simulink model "Dyn_PointMass_R2015B"  (R2015b)
settings: Solver=ode4  SolverMode=SingleTasking  StartTime=0.0  StopTime=simInit.TSIM  FixedStep=simInit.dt  MaxStep=simInit.dt  RelTol=1e-3
InitFcn:
  | close all
undefined symbols (not defined in the file): base_windspeed, constr, DE2019, DiscIntNeverNeededParam, ENVMT, Lbooth, loiterStates, params, simInit, T, winchParameter
libraries: simulink x40, simulink_extras x3, dspsigops x1
(part 2 of 5)

== system Dyn_PointMass_R2015B/WinchControl_SS_6/WinchDynamics ==
  for_tether_tot : Inport
  control_moments : Inport  Port=2
  Discrete-Time Integrator : DiscreteIntegrator  InitialCondition=winchParameter.lj_dot_init  InitialConditionSetting=State (most efficient)  SampleTime=-1  LimitOutput=on  UpperSaturationLimit=constr.winchParameter.v_max/winchParameter.radius  LowerSaturationLimit=constr.winchParameter.v_min/winchParameter.radius  ICPrevOutput=DiscIntNeverNeededParam  ICPrevScaledInput=DiscIntNeverNeededParam
  FrictionCoefficient : Gain  Gain=winchParameter.friction
  Gain{,2..6} (6 alike) : Gain  Gain=winchParameter.radius
  Gain1 : Gain  Gain=1/winchParameter.inertia
  Integrator : Integrator  InitialCondition=winchParameter.winch_angle_init
  Saturation1 : Saturate  UpperLimit=constr.winchParameter.a_max/winchParameter.radius  LowerLimit=constr.winchParameter.a_min/winchParameter.radius
  Sum : Sum  Inputs=+-+
  winch acc : Scope  NumInputPorts=2
  tether_length : Outport
  theta_dot : Outport  Port=2
  winch_acc : Outport  Port=3
  winch_vel : Outport  Port=4
  wires:
  Gain/1 -> tether_length/1
  Gain2/1 -> Sum/1
  Sum/1 -> Gain1/1
  Integrator/1 -> Gain/1  "winch_angle"
  Discrete-Time Integrator/1 -> Gain4/1, FrictionCoefficient/1, theta_dot/1, Integrator/1  "winch_angVel"
  control_moments/1 -> Sum/3
  FrictionCoefficient/1 -> Sum/2
  for_tether_tot/1 -> Gain2/1
  Gain1/1 -> Saturation1/1, Gain5/1, Gain3/1
  Saturation1/1 -> Discrete-Time Integrator/1, Gain6/1  "omega_dot"
  Gain4/1 -> winch_vel/1
  Gain3/1 -> winch_acc/1
  Gain5/1 -> winch acc/1
  Gain6/1 -> winch acc/2

== system Dyn_PointMass_R2015B/AirborneSystem/AttitudeDynamics/SecondOrderReferenceModel_alpha_a ==
  y_cmd : Inport
  Constant : Constant  Value=omega0_max
  Discrete-Time Integrator : DiscreteIntegrator  InitialConditionSetting=State (most efficient)  SampleTime=-1  LimitOutput=on  UpperSaturationLimit=y_max  LowerSaturationLimit=y_min  ICPrevOutput=DiscIntNeverNeededParam  ICPrevScaledInput=DiscIntNeverNeededParam
  Discrete-Time Integrator1 : DiscreteIntegrator  InitialConditionSetting=State (most efficient)  SampleTime=-1  LimitOutput=on  UpperSaturationLimit=yd_max  LowerSaturationLimit=yd_min  ICPrevOutput=DiscIntNeverNeededParam  ICPrevScaledInput=DiscIntNeverNeededParam
  Gain2 : Gain  Gain=2*zeta0
  Product : Product  Inputs=3
  Product1 : Product
  Saturation : Saturate  UpperLimit=y_max  LowerLimit=y_min
  Saturation1 : Saturate  UpperLimit=y2d_max  LowerLimit=y2d_min
  Sum : Sum  Inputs=|+-
  Sum1 : Sum  Inputs=|+-
  y_ref : Outport
  wires:
  Product1/1 -> Gain2/1
  Constant/1 -> Product1/2, Product/3, Product/1
  Product/1 -> Sum/1
  y_cmd/1 -> Saturation/1
  Discrete-Time Integrator1/1 -> Discrete-Time Integrator/1, Product1/1
  Sum/1 -> Saturation1/1
  Gain2/1 -> Sum/2
  Sum1/1 -> Product/2
  Saturation1/1 -> Discrete-Time Integrator1/1
  Saturation/1 -> Sum1/1
  Discrete-Time Integrator/1 -> y_ref/1, Sum1/2

== system Dyn_PointMass_R2015B/AirborneSystem/AttitudeDynamics/SecondOrderReferenceModel_mu_a ==
  y_cmd : Inport
  Constant : Constant  Value=omega0_max
  Discrete-Time Integrator : DiscreteIntegrator  InitialConditionSetting=State (most efficient)  SampleTime=-1  LimitOutput=on  UpperSaturationLimit=y_max  LowerSaturationLimit=y_min  ICPrevOutput=DiscIntNeverNeededParam  ICPrevScaledInput=DiscIntNeverNeededParam
  Discrete-Time Integrator1 : DiscreteIntegrator  InitialConditionSetting=State (most efficient)  SampleTime=-1  LimitOutput=on  UpperSaturationLimit=yd_max  LowerSaturationLimit=yd_min  ICPrevOutput=DiscIntNeverNeededParam  ICPrevScaledInput=DiscIntNeverNeededParam
  Gain2 : Gain  Gain=2*zeta0
  Product : Product  Inputs=3
  Product1 : Product
  Saturation : Saturate  UpperLimit=y_max  LowerLimit=y_min
  Saturation1 : Saturate  UpperLimit=y2d_max  LowerLimit=y2d_min
  Sum : Sum  Inputs=|+-
  Sum1 : Sum  Inputs=|+-
  y_ref : Outport
  wires:
  Product1/1 -> Gain2/1
  Constant/1 -> Product1/2, Product/3, Product/1
  Product/1 -> Sum/1
  y_cmd/1 -> Saturation/1
  Discrete-Time Integrator1/1 -> Discrete-Time Integrator/1, Product1/1
  Sum/1 -> Saturation1/1
  Gain2/1 -> Sum/2
  Sum1/1 -> Product/2
  Saturation1/1 -> Discrete-Time Integrator1/1
  Saturation/1 -> Sum1/1
  Discrete-Time Integrator/1 -> y_ref/1, Sum1/2

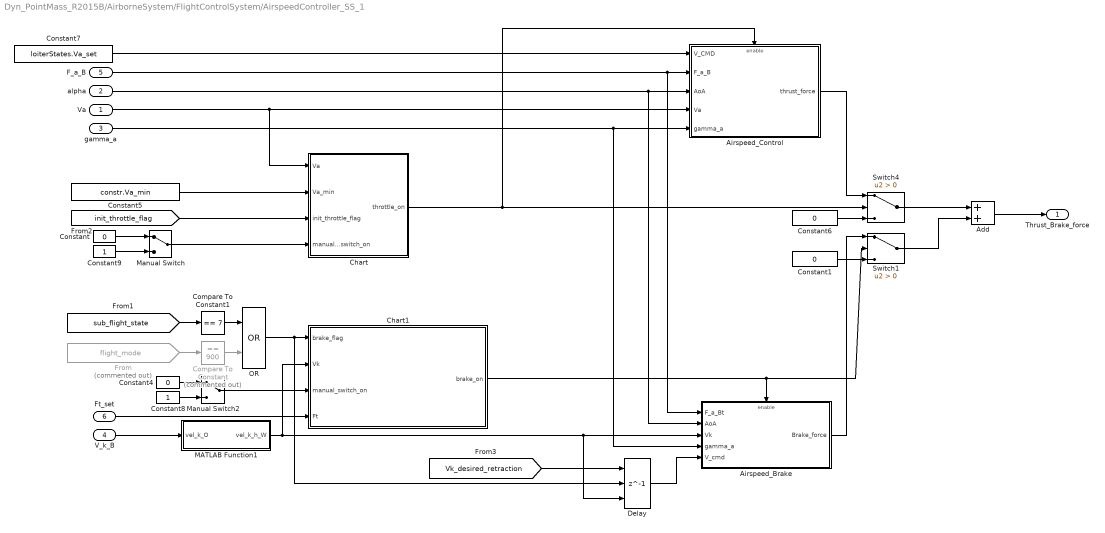
== system Dyn_PointMass_R2015B/AirborneSystem/FlightControlSystem/AirspeedController_SS_1 ==
  Va : Inport
  alpha : Inport  Port=2
  gamma_a : Inport  Port=3
  V_k_B : Inport  Port=4
  F_a_B : Inport  Port=5
  Ft_set : Inport  Port=6
  Add : Sum
  Airspeed_Brake : Subsystem
  Airspeed_Control : Subsystem
  Chart : Stateflow chart  TreatAsAtomicUnit=on
  Chart1 : Stateflow chart  TreatAsAtomicUnit=on  mask{Ft_retract=params.F_t_retraction_set*params.F_t_traction_set, Vk_min=30}
      mask prompts: Ft_retract "Retraction force"; Vk_min "Minimum Vk"
  Compare To Constant : simulink/Logic and Bit Operations/Compare To Constant  Commented=on  relop===  const=900  OutDataTypeStr=boolean
  Compare To Constant1 : simulink/Logic and Bit Operations/Compare To Constant  relop===  const=7  OutDataTypeStr=boolean
  Constant{,1,4,6} (4 alike) : Constant  Value=0
  Constant5 : Constant  Value=constr.Va_min
  Constant7 : Constant  Value=loiterStates.Va_set
  Constant8 : Constant
  Constant9 : Constant
  Delay : Delay  DelayLength=1  InitialConditionSource=Input port  ExternalReset=Rising
      settings: InputPortMap=u0,r5,p4
  From : From  Commented=on  GotoTag=flight_mode  TagVisibility=global
  MATLAB Function1 : MATLAB Function  TreatAsAtomicUnit=on
  Manual Switch : ManualSwitch
  Manual Switch2 : ManualSwitch
  OR : Logic  Operator=OR  IconShape=distinctive  AllPortsSameDT=off  OutDataTypeStr=boolean
  Switch1 : Switch  Criteria=u2 > Threshold
  Switch4 : Switch  Criteria=u2 > Threshold
  Thrust_Brake_force : Outport
  wires:
  Switch1/1 -> Add/2
  Constant1/1 -> Switch1/3
  [Vk_desired_retraction] -> Delay/1
  Compare To Constant/1 -> OR/2
  Compare To Constant1/1 -> OR/1
  MATLAB Function1/1(vel_k_h_W) -> Chart1/2(Vk), Delay/3, Airspeed_Brake/3(Vk)
  V_k_B/1 -> MATLAB Function1/1(vel_k_O)
  Delay/1 -> Airspeed_Brake/5(V_cmd)
  Constant8/1 -> Manual Switch2/2
  Constant4/1 -> Manual Switch2/1
  Add/1 -> Thrust_Brake_force/1
  From/1 -> Compare To Constant/1
  [sub_flight_state] -> Compare To Constant1/1
  OR/1 -> Chart1/1(brake_flag), Delay/2
  Manual Switch2/1 -> Chart1/3(manual_switch_on)
  Ft_set/1 -> Chart1/4(Ft)
  Airspeed_Brake/1(Brake_force) -> Switch1/1
  Chart1/1(brake_on) -> Switch1/2, Airspeed_Brake/Enable
  Airspeed_Control/1(thrust_force) -> Switch4/1
  Constant5/1 -> Chart/2(Va_min)
  Va/1 -> Chart/1(Va), Airspeed_Control/4(Va)
  Chart/1(throttle_on) -> Switch4/2, Airspeed_Control/Enable
  Constant9/1 -> Manual Switch/2
  [init_throttle_flag] -> Chart/3(init_throttle_flag)
  alpha/1 -> Airspeed_Control/3(AoA), Airspeed_Brake/2(AoA)
  Constant7/1 -> Airspeed_Control/1(V_CMD)
  Manual Switch/1 -> Chart/4(manual_switch_on)
  Constant/1 -> Manual Switch/1
  Constant6/1 -> Switch4/3
  F_a_B/1 -> Airspeed_Control/2(F_a_B), Airspeed_Brake/1(F_a_Bt)
  gamma_a/1 -> Airspeed_Control/5(gamma_a), Airspeed_Brake/4(gamma_a)
  Switch4/1 -> Add/1

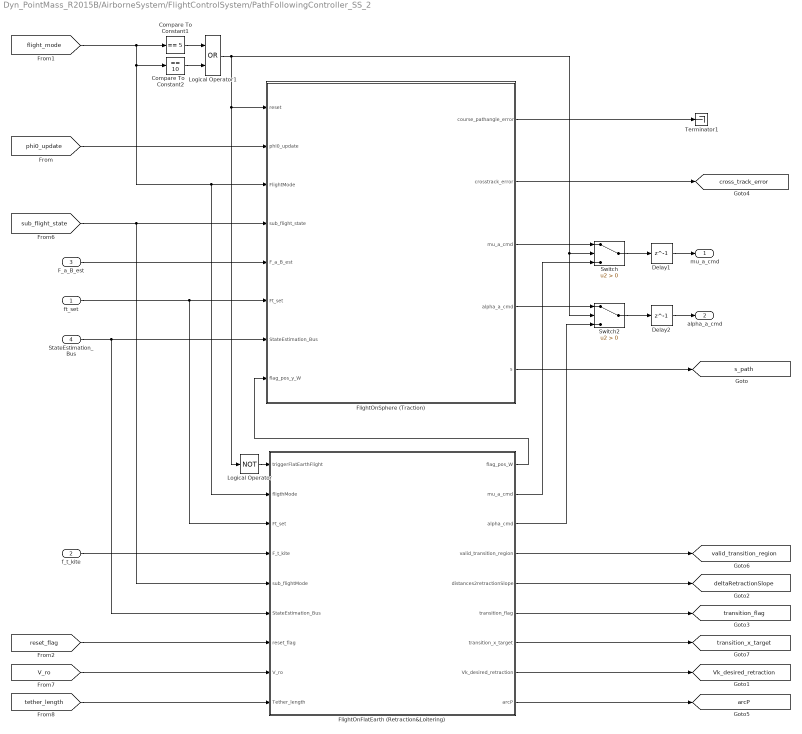
== system Dyn_PointMass_R2015B/AirborneSystem/FlightControlSystem/PathFollowingController_SS_2 ==
  ft_set : Inport
  f_t_kite : Inport  Port=2
  F_a_B_est : Inport  Port=3  PortDimensions=[3,1]
  StateEstimation_Bus : Inport  Port=4
  Compare To Constant1 : simulink/Logic and Bit Operations/Compare To Constant  relop===  const=5  OutDataTypeStr=boolean
  Compare To Constant2 : simulink/Logic and Bit Operations/Compare To Constant  relop===  const=10  OutDataTypeStr=boolean
  Delay1 : Delay  DelayLength=1
  Delay2 : Delay  DelayLength=1
  FlightOnFlatEarth (Retraction&Loitering) : Subsystem
  FlightOnSphere (Traction) : Subsystem
  Logical Operator : Logic  Operator=NOT  AllPortsSameDT=off  OutDataTypeStr=boolean
  Logical Operator1 : Logic  Operator=OR  AllPortsSameDT=off  OutDataTypeStr=boolean
  Switch : Switch  Criteria=u2 > Threshold
  Switch2 : Switch  Criteria=u2 > Threshold
  Terminator1 : Terminator
  mu_a_cmd : Outport  PortDimensions=1
  alpha_a_cmd : Outport  Port=2  PortDimensions=1
  tag scope: Vk_desired_retraction=global, arcP=global, cross_track_error=global, deltaRetractionSlope=global, s_path=global, transition_flag=global, transition_x_target=global, valid_transition_region=global
  wires:
  FlightOnFlatEarth (Retraction&Loitering)/9(arcP) -> [arcP]
  [sub_flight_state] -> FlightOnSphere (Traction)/4(sub_flight_state), FlightOnFlatEarth (Retraction&Loitering)/5(sub_flightMode)
  [tether_length] -> FlightOnFlatEarth (Retraction&Loitering)/9(Tether_length)
  [V_ro] -> FlightOnFlatEarth (Retraction&Loitering)/8(V_ro)
  FlightOnFlatEarth (Retraction&Loitering)/8(Vk_desired_retraction) -> [Vk_desired_retraction]
  FlightOnFlatEarth (Retraction&Loitering)/7(transition_x_target) -> [transition_x_target]
  FlightOnFlatEarth (Retraction&Loitering)/1(flag_pos_W) -> FlightOnSphere (Traction)/8(flag_pos_y_W)
  FlightOnFlatEarth (Retraction&Loitering)/5(distances2retractionSlope) -> [deltaRetractionSlope]
  [reset_flag] -> FlightOnFlatEarth (Retraction&Loitering)/7(reset_flag)
  FlightOnFlatEarth (Retraction&Loitering)/6(transition_flag) -> [transition_flag]
  [phi0_update] -> FlightOnSphere (Traction)/2(phi0_update)
  FlightOnSphere (Traction)/5(s) -> [s_path]
  Compare To Constant2/1 -> Logical Operator1/2
  Compare To Constant1/1 -> Logical Operator1/1
  [flight_mode] -> Compare To Constant2/1, FlightOnSphere (Traction)/3(FlightMode), FlightOnFlatEarth (Retraction&Loitering)/2(fligthMode), Compare To Constant1/1
  FlightOnSphere (Traction)/2(crosstrack_error) -> [cross_track_error]
  FlightOnSphere (Traction)/1(course_pathangle_error) -> Terminator1/1
  FlightOnSphere (Traction)/3(mu_a_cmd) -> Switch/1
  FlightOnSphere (Traction)/4(alpha_a_cmd) -> Switch2/1
  F_a_B_est/1 -> FlightOnSphere (Traction)/5(F_a_B_est)
  f_t_kite/1 -> FlightOnFlatEarth (Retraction&Loitering)/4(F_t_kite)
  Switch2/1 -> Delay2/1
  Switch/1 -> Delay1/1
  Delay1/1 -> mu_a_cmd/1
  Delay2/1 -> alpha_a_cmd/1
  ft_set/1 -> FlightOnSphere (Traction)/6(Ft_set), FlightOnFlatEarth (Retraction&Loitering)/3(Ft_set)
  Logical Operator/1 -> FlightOnFlatEarth (Retraction&Loitering)/1(triggerFlatEarthFlight)
  FlightOnFlatEarth (Retraction&Loitering)/2(mu_a_cmd) -> Switch/3
  FlightOnFlatEarth (Retraction&Loitering)/3(alpha_cmd) -> Switch2/3
  FlightOnFlatEarth (Retraction&Loitering)/4(valid_transition_region) -> [valid_transition_region]
  Logical Operator1/1 -> Switch2/2, Switch/2, Logical Operator/1, FlightOnSphere (Traction)/1(reset)
  StateEstimation_Bus/1 -> FlightOnFlatEarth (Retraction&Loitering)/6(StateEstimation_Bus), FlightOnSphere (Traction)/7(StateEstimation_Bus)

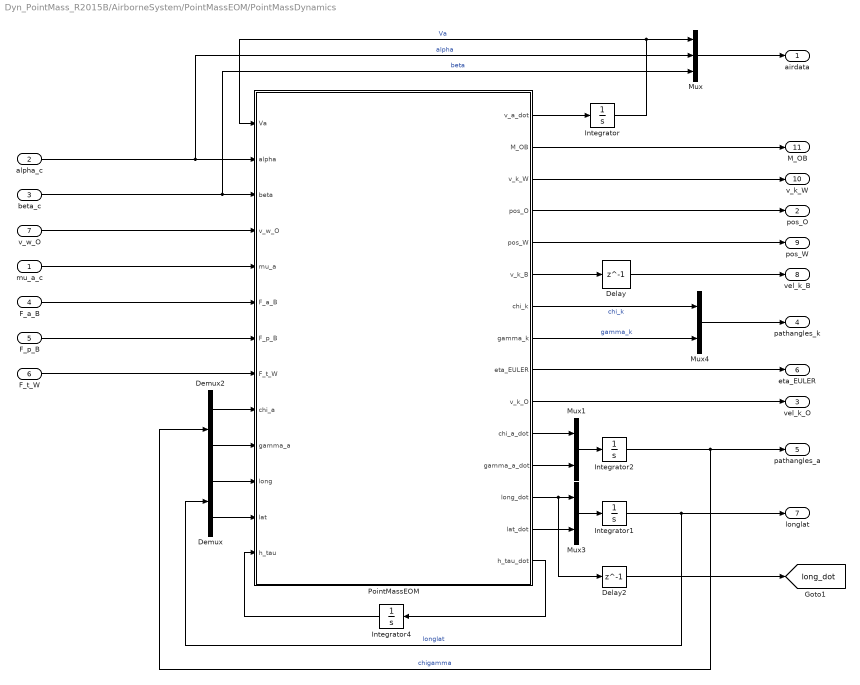
== system Dyn_PointMass_R2015B/AirborneSystem/PointMassEOM/PointMassDynamics ==
  mu_a_c : Inport
  alpha_c : Inport  Port=2
  beta_c : Inport  Port=3
  F_a_B : Inport  Port=4  PortDimensions=[3,1]
  F_p_B : Inport  Port=5  PortDimensions=[3,1]
  F_t_W : Inport  Port=6  PortDimensions=[3,1]
  v_w_O : Inport  Port=7
  Delay : Delay  DelayLength=1  InitialCondition=simInit.vel_B_init
  Delay2 : Delay  DelayLength=1
  Demux : Demux  Outputs=2
  Demux2 : Demux  Outputs=2
  Integrator : Integrator  InitialCondition=simInit.vel_B_init(1)
  Integrator1 : Integrator  InitialCondition=[simInit.long_init;simInit.lat_init]  WrapState=on
  Integrator2 : Integrator  InitialCondition=zeros(2,1)  WrapState=on
  Integrator4 : Integrator  InitialCondition=norm(simInit.pos_O_init)
  Mux : Mux  Inputs=3
  Mux1 : Mux  Inputs=2
  Mux3 : Mux  Inputs=2
  Mux4 : Mux  Inputs=2
  PointMassEOM : MATLAB Function  TreatAsAtomicUnit=on
  airdata : Outport  PortDimensions=3
  pos_O : Outport  Port=2  PortDimensions=[3,1]
  vel_k_O : Outport  Port=3  PortDimensions=[3,1]
  pathangles_k : Outport  Port=4  PortDimensions=2
  pathangles_a : Outport  Port=5  PortDimensions=2
  eta_EULER : Outport  Port=6  PortDimensions=[3,1]
  longlat : Outport  Port=7  PortDimensions=2
  vel_k_B : Outport  Port=8  PortDimensions=[3,1]
  pos_W : Outport  Port=9  PortDimensions=[3,1]
  v_k_W : Outport  Port=10  PortDimensions=[3,1]
  M_OB : Outport  Port=11  PortDimensions=[3,3]
  tag scope: long_dot=global
  wires:
  F_p_B/1 -> PointMassEOM/7(F_p_B)
  mu_a_c/1 -> PointMassEOM/5(mu_a)
  PointMassEOM/7(chi_k) -> Mux4/1  "chi_k"
  F_a_B/1 -> PointMassEOM/6(F_a_B)
  Integrator/1 -> PointMassEOM/1(Va), Mux/1  "Va"
  PointMassEOM/8(gamma_k) -> Mux4/2  "gamma_k"
  PointMassEOM/12(gamma_a_dot) -> Mux1/2
  Integrator4/1 -> PointMassEOM/13(h_tau)
  PointMassEOM/14(lat_dot) -> Mux3/2
  PointMassEOM/11(chi_a_dot) -> Mux1/1
  PointMassEOM/15(h_tau_dot) -> Integrator4/1
  PointMassEOM/1(v_a_dot) -> Integrator/1
  Demux2/2 -> PointMassEOM/10(gamma_a)
  v_w_O/1 -> PointMassEOM/4(v_w_O)
  PointMassEOM/9(eta_EULER) -> eta_EULER/1
  Mux/1 -> airdata/1
  alpha_c/1 -> Mux/2, PointMassEOM/2(alpha)  "alpha"
  beta_c/1 -> Mux/3, PointMassEOM/3(beta)  "beta"
  PointMassEOM/10(v_k_O) -> vel_k_O/1
  PointMassEOM/6(v_k_B) -> Delay/1
  PointMassEOM/5(pos_W) -> pos_W/1
  PointMassEOM/4(pos_O) -> pos_O/1
  Demux2/1 -> PointMassEOM/9(chi_a)
  PointMassEOM/3(v_k_W) -> v_k_W/1
  PointMassEOM/2(M_OB) -> M_OB/1
  PointMassEOM/13(long_dot) -> Mux3/1, Delay2/1
  Mux3/1 -> Integrator1/1
  Delay2/1 -> [long_dot]
  Integrator1/1 -> longlat/1, Demux/1  "longlat"
  Demux/1 -> PointMassEOM/11(long)
  Demux/2 -> PointMassEOM/12(lat)
  Mux1/1 -> Integrator2/1
  Integrator2/1 -> pathangles_a/1, Demux2/1  "chigamma"
  F_t_W/1 -> PointMassEOM/8(F_t_W)
  Delay/1 -> vel_k_B/1
  Mux4/1 -> pathangles_k/1

== system Dyn_PointMass_R2015B/Environment_SS_3/Windshear/Wind Shear Model ==
  Altitude : Inport
  DCM : Inport  Port=2  PortDimensions=[3 3]
  Degrees to Radians : simulink_extras/Transformations/Degrees to Radians
  Disallow CGS : UnitConfiguration  UnitSystemsStr=English,SI,SI (extended)  AllowAllUnitSystems=off
  Mux : Mux  Inputs=3
  Reshape1 : Reshape
  SinCos : Trigonometry  Operator=sincos
  Transform from Inertial to Body axes : Product  Inputs=**  Multiplication=Matrix(*)  SaturateOnIntegerOverflow=on  InputSameDT=on  OutDataTypeStr=Inherit: Same as first input
  Wdeg1 : Constant  Value=0  OutDataTypeStr=Inherit: Inherit via back propagation
  Wind Direction : Constant  Value=ENVMT.windDirection_rad*180/pi  OutDataTypeStr=Inherit: Inherit via back propagation
  Wind speed at reference height : Gain  Gain=-base_windspeed  SaturateOnIntegerOverflow=on  OutDataTypeStr=Inherit: Same as input  ParamDataTypeStr=Inherit: Same as input
  wind_field_calc : Subsystem
  Mean Wind : Outport
  wires:
  Reshape1/1 -> Mean Wind/1
  wind_field_calc/1(Windspeed_altitude) -> Transform from Inertial to Body axes/2
  Degrees to Radians/1 -> SinCos/1
  Wind speed at reference height/1 -> wind_field_calc/2(Base_windspeed)
  DCM/1 -> Transform from Inertial to Body axes/1
  Mux/1 -> Wind speed at reference height/1
  Wdeg1/1 -> Mux/3  "Wz"
  SinCos/1 -> Mux/2  "Wy"
  SinCos/2 -> Mux/1  "Wx"
  Wind Direction/1 -> Degrees to Radians/1
  Transform from Inertial to Body axes/1 -> Reshape1/1
  Altitude/1 -> wind_field_calc/1(Altitude)

== system Dyn_PointMass_R2015B/Environment_SS_3/wind_field_calc/Length Conversion ==
  in : Inport
  Unit Conversion : UnitConversion
  out : Outport
  wires:
  Unit Conversion/1 -> out/1
  in/1 -> Unit Conversion/1

== system Dyn_PointMass_R2015B/WinchControl_SS_6/PureTorqueControl/PI-ForceController ==
  RetractionFlag : Inport
  controlDeficitDue2Sat : Inport  Port=2
  e_Ft : Inport  Port=3
  Abs : Abs
  Compare To Constant : simulink/Logic and Bit Operations/Compare To Constant  relop=>=  const=1e-3  OutDataTypeStr=boolean
  Constant2 : Constant  Value=0
  Gain8 : Gain  Gain=params.ki_winch
  Gain9 : Gain  Gain=params.kp_winch
  Integrator : Integrator
  Logical Operator : Logic  Operator=OR  AllPortsSameDT=off  OutDataTypeStr=boolean
  Sum8 : Sum
  Switch : Switch  Criteria=u2 > Threshold
  TorqueCmd : Outport
  wires:
  Sum8/1 -> TorqueCmd/1
  Switch/1 -> Integrator/1
  Constant2/1 -> Switch/1
  Gain9/1 -> Sum8/2
  Gain8/1 -> Switch/3
  Compare To Constant/1 -> Logical Operator/2
  Integrator/1 -> Sum8/1
  Abs/1 -> Compare To Constant/1
  e_Ft/1 -> Gain8/1, Gain9/1
  controlDeficitDue2Sat/1 -> Abs/1
  RetractionFlag/1 -> Logical Operator/1
  Logical Operator/1 -> Switch/2

== system Dyn_PointMass_R2015B/AirborneSystem/FlightControlSystem/AirspeedController_SS_1/Airspeed_Brake ==
  F_a_Bt : Inport  PortDimensions=[3,1]
  AoA : Inport  Port=2
  Vk : Inport  Port=3
  gamma_a : Inport  Port=4
  V_cmd : Inport  Port=5
  Enable : EnablePort
  Delay1 : Delay  DelayLength=1  InitialConditionSource=Input port  InitialCondition=zeros(3,1)
      settings: InputPortMap=u0,p4
  Discrete-Time Integrator : DiscreteIntegrator  InitialConditionSetting=State (most efficient)  SampleTime=-1  ICPrevOutput=DiscIntNeverNeededParam  ICPrevScaledInput=DiscIntNeverNeededParam
  FeedforwardPart : MATLAB Function  TreatAsAtomicUnit=on
  Gain3 : Gain  Gain=params.Kp_brake
  Gain4 : Gain  Gain=params.Ki_brake
  MATLAB Function : MATLAB Function  TreatAsAtomicUnit=on
  Saturation : Saturate  UpperLimit=0  LowerLimit=-inf  LinearizeAsGain=off
  Scope : Scope  NumInputPorts=3
  Scope1 : Scope
  Subsystem : Subsystem
  Sum1 : Sum
  Sum2 : Sum  Inputs=|+-
  Sum3 : Sum  Inputs=-+|
  hedging : MATLAB Function  TreatAsAtomicUnit=on
  Brake_force : Outport
  wires:
  AoA/1 -> MATLAB Function/2(AoA)
  MATLAB Function/1(Drag) -> FeedforwardPart/3(Drag_force), hedging/1(Drag_force)
  F_a_Bt/1 -> MATLAB Function/1(F_a_B)
  Sum2/1 -> Subsystem/2(v_h)
  hedging/1(nu_V) -> Sum2/2
  FeedforwardPart/1(BF) -> Saturation/1
  Saturation/1 -> Brake_force/1, Scope1/1, hedging/3(BF)
  Sum1/1 -> Sum2/1, FeedforwardPart/2(nu_V)
  Subsystem/1(V_k_ref) -> Scope/3, Sum3/2
  gamma_a/1 -> hedging/2(gamma), FeedforwardPart/1(gamma)
  Sum3/1 -> Gain4/1, Gain3/1
  Gain3/1 -> Sum1/1
  Discrete-Time Integrator/1 -> Sum1/2
  Gain4/1 -> Discrete-Time Integrator/1
  V_cmd/1 -> Scope/1, Subsystem/1(V_cmd)
  Delay1/1 -> Subsystem/3(Initial), Delay1/1
  Vk/1 -> Delay1/2, Sum3/1, Scope/2

== system Dyn_PointMass_R2015B/AirborneSystem/FlightControlSystem/AirspeedController_SS_1/Airspeed_Control ==
  V_CMD : Inport
  F_a_B : Inport  Port=2  PortDimensions=[3,1]
  AoA : Inport  Port=3
  Va : Inport  Port=4
  gamma_a : Inport  Port=5
  Enable : EnablePort
  Discrete-Time Integrator : DiscreteIntegrator  InitialConditionSetting=State (most efficient)  SampleTime=-1  ICPrevOutput=DiscIntNeverNeededParam  ICPrevScaledInput=DiscIntNeverNeededParam
  FeedforwardPart : MATLAB Function  TreatAsAtomicUnit=on
  Gain3 : Gain  Gain=params.kp_speed_control
  Gain4 : Gain  Gain=params.ki_speed_control
  MATLAB Function : MATLAB Function  TreatAsAtomicUnit=on
  Saturation : Saturate  UpperLimit=inf  LowerLimit=0  LinearizeAsGain=off
  Scope : Scope  NumInputPorts=3
  Subsystem : Subsystem
  Sum : Sum  Inputs=-+|
  Sum1 : Sum  Inputs=+++
  Sum2 : Sum  Inputs=|+-
  hedging : MATLAB Function  TreatAsAtomicUnit=on
  thrust_force : Outport
  wires:
  AoA/1 -> MATLAB Function/2(AoA)
  MATLAB Function/1(Drag) -> hedging/1(Drag_force), FeedforwardPart/3(Drag_force)
  F_a_B/1 -> MATLAB Function/1(F_a_B)
  Sum2/1 -> Subsystem/2(v_h)
  hedging/1(nu_V) -> Sum2/2
  FeedforwardPart/1(T) -> Saturation/1
  Saturation/1 -> thrust_force/1, hedging/3(T)
  Subsystem/1(V_k_ref_dot) -> Sum1/1
  Sum1/1 -> Sum2/1, FeedforwardPart/2(nu_V)
  Subsystem/2(V_k_ref) -> Sum/2, Scope/3
  gamma_a/1 -> hedging/2(gamma), FeedforwardPart/1(gamma)
  V_CMD/1 -> Subsystem/1(V_cmd), Scope/1
  Sum/1 -> Gain4/1, Gain3/1
  Va/1 -> Scope/2, Sum/1
  Gain3/1 -> Sum1/2
  Discrete-Time Integrator/1 -> Sum1/3
  Gain4/1 -> Discrete-Time Integrator/1

== system Dyn_PointMass_R2015B/AirborneSystem/FlightControlSystem/PathFollowingController_SS_2/FlightOnFlatEarth (Retraction&Loitering) ==
  triggerFlatEarthFlight : Inport
  fligthMode : Inport  Port=2
  Ft_set : Inport  Port=3
  F_t_kite : Inport  Port=4
  sub_flightMode : Inport  Port=5
  StateEstimation_Bus : Inport  Port=6
  reset_flag : Inport  Port=7
  V_ro : Inport  Port=8
  Tether_length : Inport  Port=9
  CalculateAttitudeCmds : Subsystem
  GuidanceFlatEarth : Subsystem
  flag_pos_W : Outport
  mu_a_cmd : Outport  Port=2
  alpha_cmd : Outport  Port=3
  valid_transition_region : Outport  Port=4
  distances2retractionSlope : Outport  Port=5
  transition_flag : Outport  Port=6
  transition_x_target : Outport  Port=7
  Vk_desired_retraction : Outport  Port=8
  arcP : Outport  Port=9
  wires:
  StateEstimation_Bus/1 -> CalculateAttitudeCmds/7(StateEstimation_Bus), GuidanceFlatEarth/2(StateEstimation_Bus)
  CalculateAttitudeCmds/1(mu_a_cmd) -> mu_a_cmd/1
  Ft_set/1 -> CalculateAttitudeCmds/3(Ft_set)
  CalculateAttitudeCmds/2(alpha_cmd) -> alpha_cmd/1
  fligthMode/1 -> CalculateAttitudeCmds/6(flightMode), GuidanceFlatEarth/1(flightMode)
  triggerFlatEarthFlight/1 -> GuidanceFlatEarth/Enable, CalculateAttitudeCmds/1(flight_on_flatearth_flag)
  GuidanceFlatEarth/3(valid_transition_region) -> valid_transition_region/1
  F_t_kite/1 -> CalculateAttitudeCmds/4(F_t_kite)
  GuidanceFlatEarth/1(distances2slope) -> distances2retractionSlope/1
  GuidanceFlatEarth/2(course_path) -> CalculateAttitudeCmds/2(pathangles_k_cmd)
  sub_flightMode/1 -> CalculateAttitudeCmds/5(sub_flightMode)
  GuidanceFlatEarth/4(transition_flag) -> transition_flag/1
  reset_flag/1 -> GuidanceFlatEarth/3(reset_flat)
  GuidanceFlatEarth/5(flag_pos_W) -> flag_pos_W/1
  GuidanceFlatEarth/6(transition_x_target) -> transition_x_target/1
  GuidanceFlatEarth/7(Vk_desired_retraction) -> Vk_desired_retraction/1
  V_ro/1 -> GuidanceFlatEarth/4(V_ro)
  Tether_length/1 -> GuidanceFlatEarth/5(Tether_length)
  GuidanceFlatEarth/8(arcP) -> arcP/1

== system Dyn_PointMass_R2015B/AirborneSystem/FlightControlSystem/PathFollowingController_SS_2/FlightOnSphere (Traction) ==
  reset : Inport
  phi0_update : Inport  Port=2
  FlightMode : Inport  Port=3  PortDimensions=1
  sub_flight_state : Inport  Port=4
  F_a_B_est : Inport  Port=5  PortDimensions=[3,1]
  Ft_set : Inport  Port=6
  StateEstimation_Bus : Inport  Port=7
  flag_pos_y_W : Inport  Port=8
  Compare To Constant1 : simulink/Logic and Bit Operations/Compare To Constant  Commented=on  relop===  const=5  OutDataTypeStr=boolean
  Compare To Constant2 : simulink/Logic and Bit Operations/Compare To Constant  Commented=on  relop===  const=1  OutDataTypeStr=boolean
  Constant : Constant  Value=Lbooth.init_sol
  FlightPathLoopTraction : Subsystem
  Logical Operator : Logic  Commented=on  Operator=OR  AllPortsSameDT=off  OutDataTypeStr=boolean
  Navigator : Subsystem
  Pcontroller_ChiGamma_Traction : Subsystem
  Sample and Hold : dspsigops/Sample and Hold  Commented=on  trig=Rising edge  initCond=0  latchinput=off
  Select_init_sol_for_pathfollowing : Stateflow chart  TreatAsAtomicUnit=on
  Sum : Sum  Inputs=|++
  Sum1 : Sum  Inputs=|++
  course_pathangle_error : Outport
  crosstrack_error : Outport  Port=2
  mu_a_cmd : Outport  Port=3  PortDimensions=1
  alpha_a_cmd : Outport  Port=4  PortDimensions=1
  s : Outport  Port=5
  wires:
  FlightPathLoopTraction/1(mu_a_c_traction) -> mu_a_cmd/1
  Navigator/5(course_pathangle_error) -> Pcontroller_ChiGamma_Traction/1(course_pathangle_error), course_pathangle_error/1
  Navigator/3(crosstrack_error) -> crosstrack_error/1
  FlightPathLoopTraction/2(alpha_rq) -> alpha_a_cmd/1
  F_a_B_est/1 -> FlightPathLoopTraction/2(F_a_B_est)
  Ft_set/1 -> FlightPathLoopTraction/1(Ft_set)
  StateEstimation_Bus/1 -> FlightPathLoopTraction/3(StateEstimation_Bus), Navigator/4(StateEstimation_Bus)
  Navigator/4(s) -> s/1
  phi0_update/1 -> Navigator/1(phi0_update)
  reset/1 -> Navigator/Enable, FlightPathLoopTraction/Enable
  Navigator/1(chi_k_dot) -> Sum/1
  Navigator/2(gamma_k_dot) -> Sum1/1
  Select_init_sol_for_pathfollowing/1(sol_init) -> Navigator/5(init_value)
  Constant/1 -> Select_init_sol_for_pathfollowing/1(x)
  Sum1/1 -> FlightPathLoopTraction/5(nu_gamma)
  Sum/1 -> FlightPathLoopTraction/4(nu_chi)
  FlightMode/1 -> Navigator/3(flight_mode), Sample and Hold/1, Compare To Constant2/1, Compare To Constant1/1, Select_init_sol_for_pathfollowing/2(fm)
  flag_pos_y_W/1 -> Select_init_sol_for_pathfollowing/3(flag_pos_y_W)
  Pcontroller_ChiGamma_Traction/1(Chi_cntr) -> Sum/2
  Pcontroller_ChiGamma_Traction/2(Gamma_cntr) -> Sum1/2
  Compare To Constant2/1 -> Logical Operator/1
  Compare To Constant1/1 -> Logical Operator/2
  Logical Operator/1 -> Sample and Hold/Trigger
  Sample and Hold/1 -> Navigator/6(fm_mem)
  sub_flight_state/1 -> Navigator/2(sub_flight_state)

== system Dyn_PointMass_R2015B/Environment_SS_3/Windshear/Wind Shear Model/wind_field_calc ==
  Altitude : Inport
  Base_windspeed : Inport  Port=2
  1-D Lookup Table : Lookup_n-D  NumberOfTableDimensions=1  BreakpointsForDimension1=ENVMT.wind_height  Table=ENVMT.wind_data  InternalRulePriority=Speed  RndMeth=Simplest  InputSameDT=on
  3ft-->inf : Saturate  Commented=on  UpperLimit=inf  LowerLimit=3
  Length Conversion : Subsystem  Commented=on
  Manual Switch : ManualSwitch  CurrentSetting=0
  Product : Product  Commented=on  Inputs=*/  SaturateOnIntegerOverflow=on  InputSameDT=on  OutDataTypeStr=Inherit: Same as first input
  Product1 : Product  Commented=on  SaturateOnIntegerOverflow=on  InputSameDT=on  OutDataTypeStr=Inherit: Same as first input
  Product2 : Product  SaturateOnIntegerOverflow=on  InputSameDT=on  OutDataTypeStr=Inherit: Same as first input
  Reshape : Reshape  OutputDimensionality=Column vector (2-D)
  Saturation : Saturate  UpperLimit=ENVMT.height_max  LowerLimit=ENVMT.wind_height(1)
  h/z0 : Gain  Commented=on  Gain=1/0.15  SaturateOnIntegerOverflow=on  OutDataTypeStr=Inherit: Same as input  ParamDataTypeStr=Inherit: Same as input
  ln(h/z0) : Math  Commented=on  Operator=log  SaturateOnIntegerOverflow=on
  ln(ref_height/z0) : Math  Commented=on  Operator=log  SaturateOnIntegerOverflow=on
  ref_height/z0 [ft] : Constant  Commented=on  Value=20/0.15  OutDataTypeStr=Inherit: Inherit via back propagation
  Windspeed_altitude : Outport
  wires:
  Altitude/1 -> Saturation/1, Length Conversion/1(in)
  ref_height/z0 [ft]/1 -> ln(ref_height/z0)/1
  h/z0/1 -> ln(h/z0)/1
  Product/1 -> Product1/1
  Manual Switch/1 -> Reshape/1
  Saturation/1 -> 1-D Lookup Table/1  "ijmuiden"
  Base_windspeed/1 -> Product2/2, Product1/2
  Product1/1 -> Manual Switch/1  "log-law"
  Length Conversion/1(out) -> 3ft-->inf/1
  ln(h/z0)/1 -> Product/1
  Reshape/1 -> Windspeed_altitude/1
  1-D Lookup Table/1 -> Product2/1
  ln(ref_height/z0)/1 -> Product/2
  Product2/1 -> Manual Switch/2  "referencce location"
  3ft-->inf/1 -> h/z0/1

== system Dyn_PointMass_R2015B/AirborneSystem/FlightControlSystem/AirspeedController_SS_1/Airspeed_Brake/Subsystem ==
  V_cmd : Inport
  v_h : Inport  Port=2
  Initial : Inport  Port=3
  Discrete-Time Integrator1 : DiscreteIntegrator  InitialConditionSource=external  InitialCondition=norm(simInit.vel_B_init)  InitialConditionSetting=State (most efficient)  SampleTime=-1  LimitOutput=on  UpperSaturationLimit=120  LowerSaturationLimit=0  ICPrevOutput=DiscIntNeverNeededParam  ICPrevScaledInput=DiscIntNeverNeededParam
  Gain2 : Gain  Gain=params.w0SpeedControl  Multiplication=Matrix(K*u)
  Sum1 : Sum  Inputs=|+-
  Sum2 : Sum  Inputs=|+-
  V_k_ref : Outport
  wires:
  Gain2/1 -> Sum1/1
  v_h/1 -> Sum1/2
  Sum1/1 -> Discrete-Time Integrator1/1
  V_cmd/1 -> Sum2/1
  Sum2/1 -> Gain2/1
  Discrete-Time Integrator1/1 -> Sum2/2, V_k_ref/1
  Initial/1 -> Discrete-Time Integrator1/2

== system Dyn_PointMass_R2015B/AirborneSystem/FlightControlSystem/AirspeedController_SS_1/Airspeed_Control/Subsystem ==
  V_cmd : Inport
  v_h : Inport  Port=2
  Discrete-Time Integrator1 : DiscreteIntegrator  InitialCondition=norm(simInit.vel_B_init)  InitialConditionSetting=State (most efficient)  SampleTime=-1  LimitOutput=on  UpperSaturationLimit=120  LowerSaturationLimit=0  ICPrevOutput=DiscIntNeverNeededParam  ICPrevScaledInput=DiscIntNeverNeededParam
  Gain2 : Gain  Gain=params.w0SpeedControl  Multiplication=Matrix(K*u)
  Sum1 : Sum  Inputs=|+-
  Sum2 : Sum  Inputs=|+-
  V_k_ref_dot : Outport
  V_k_ref : Outport  Port=2
  wires:
  Gain2/1 -> Sum1/1, V_k_ref_dot/1
  v_h/1 -> Sum1/2
  Sum1/1 -> Discrete-Time Integrator1/1
  V_cmd/1 -> Sum2/1
  Sum2/1 -> Gain2/1
  Discrete-Time Integrator1/1 -> V_k_ref/1, Sum2/2

== system Dyn_PointMass_R2015B/AirborneSystem/FlightControlSystem/PathFollowingController_SS_2/FlightOnFlatEarth (Retraction&Loitering)/CalculateAttitudeCmds ==
  flight_on_flatearth_flag : Inport
  pathangles_k_cmd : Inport  Port=2
  Ft_set : Inport  Port=3
  F_t_kite : Inport  Port=4
  sub_flightMode : Inport  Port=5
  flightMode : Inport  Port=6
  StateEstimation_Bus : Inport  Port=7
  Demux : Demux  Outputs=3
  FlightPathLoopRetraction_Aerodynamic : Subsystem
  Mux1 : Mux  Inputs=3
  Signal Specification : SignalSpecification  Dimensions=[3,1]
  Terminator2 : Terminator
  mu_a_cmd : Outport
  alpha_cmd : Outport  Port=2
  wires:
  StateEstimation_Bus/1 -> FlightPathLoopRetraction_Aerodynamic/4(StateEstimation_Bus)
  Demux/3 -> Terminator2/1
  Demux/2 -> alpha_cmd/1
  flight_on_flatearth_flag/1 -> FlightPathLoopRetraction_Aerodynamic/Enable
  FlightPathLoopRetraction_Aerodynamic/2(alpha_a_cmd) -> Mux1/2
  flightMode/1 -> FlightPathLoopRetraction_Aerodynamic/1(flight_mode)
  Signal Specification/1 -> Demux/1
  Demux/1 -> mu_a_cmd/1
  Mux1/1 -> Signal Specification/1
  F_t_kite/1 -> FlightPathLoopRetraction_Aerodynamic/3(F_t_kite)
  FlightPathLoopRetraction_Aerodynamic/1(mu_a_cmd) -> Mux1/1
  Ft_set/1 -> FlightPathLoopRetraction_Aerodynamic/2(F_t_set)
  FlightPathLoopRetraction_Aerodynamic/3(beta_a_cmd) -> Mux1/3
  pathangles_k_cmd/1 -> FlightPathLoopRetraction_Aerodynamic/5(kinematic_path_cmd)
  sub_flightMode/1 -> FlightPathLoopRetraction_Aerodynamic/6(sub_flightMode)

== system Dyn_PointMass_R2015B/AirborneSystem/FlightControlSystem/PathFollowingController_SS_2/FlightOnFlatEarth (Retraction&Loitering)/GuidanceFlatEarth ==
  flightMode : Inport
  StateEstimation_Bus : Inport  Port=2
  reset_flat : Inport  Port=3
  V_ro : Inport  Port=4
  Tether_length : Inport  Port=5
  Enable : EnablePort
  Bus Selector : BusSelector  OutputSignals=pos_G_O_m,vel_K_O_mDs,pathangles_k,pos_G_W
  Compare To Constant : simulink/Logic and Bit Operations/Compare To Constant  relop===  const=6  OutDataTypeStr=boolean
  Compare To Constant2 : simulink/Logic and Bit Operations/Compare To Constant  relop===  const=6  OutDataTypeStr=boolean
  LoiteringGuidance : Subsystem
  Retraction_Nav : Subsystem
  Switch1 : Switch  Criteria=u2 > Threshold
  distances2slope : Outport
  course_path : Outport  Port=2
  valid_transition_region : Outport  Port=3
  transition_flag : Outport  Port=4
  flag_pos_W : Outport  Port=5
  transition_x_target : Outport  Port=6
  Vk_desired_retraction : Outport  Port=7
  arcP : Outport  Port=8
  wires:
  Bus Selector/1 -> Retraction_Nav/1(pos_O), LoiteringGuidance/2(pos_G_O_m)  "<pos_G_O_m>"
  StateEstimation_Bus/1 -> Bus Selector/1
  Bus Selector/2 -> Retraction_Nav/2(vel_k_O), LoiteringGuidance/3(vel_K_O_mDs)  "<vel_K_O_mDs>"
  Compare To Constant2/1 -> Retraction_Nav/Enable
  Switch1/1 -> course_path/1
  Compare To Constant/1 -> Switch1/2
  Retraction_Nav/1(distances2slope) -> distances2slope/1
  Retraction_Nav/7(path_k_cmds) -> Switch1/1
  flightMode/1 -> LoiteringGuidance/1(flightMode), Compare To Constant/1, Compare To Constant2/1
  Bus Selector/3 -> LoiteringGuidance/4(pathangles_k)  "<pathangles_k>"
  LoiteringGuidance/1(path_k_cmds) -> Switch1/3
  LoiteringGuidance/2(valid_transition_region) -> valid_transition_region/1
  Retraction_Nav/2(transition_flag) -> transition_flag/1
  reset_flat/1 -> LoiteringGuidance/6(reset_flag)
  Bus Selector/4 -> LoiteringGuidance/5(pos_W)  "<pos_G_W>"
  Retraction_Nav/3(flag_pos_y_W) -> flag_pos_W/1
  Retraction_Nav/4(transition_x_target) -> transition_x_target/1
  Retraction_Nav/5(Vk_desired_retraction) -> Vk_desired_retraction/1
  V_ro/1 -> Retraction_Nav/3(V_ro)
  Tether_length/1 -> Retraction_Nav/4(Tether_length)
  Retraction_Nav/6(arcP) -> arcP/1

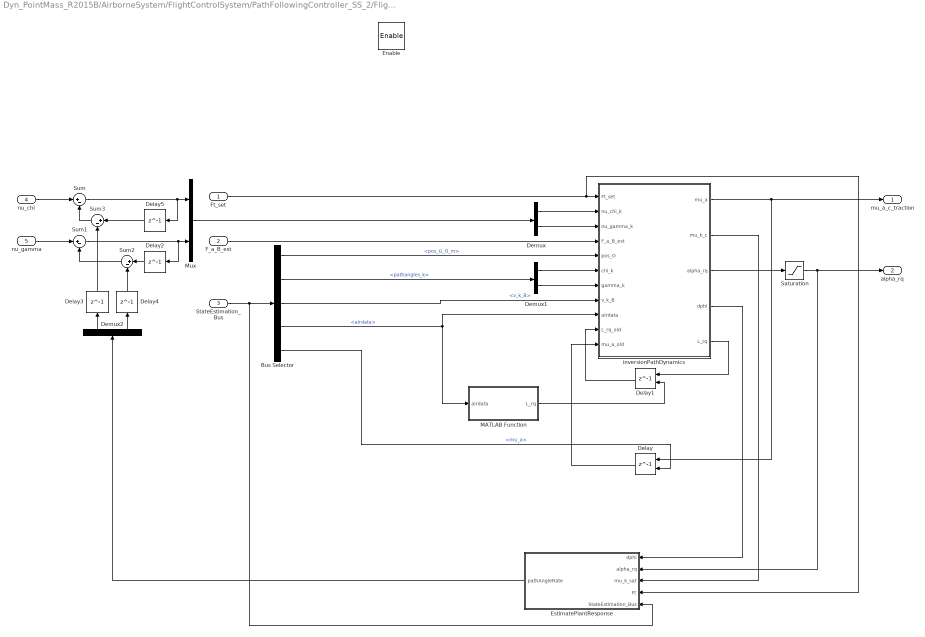
== system Dyn_PointMass_R2015B/AirborneSystem/FlightControlSystem/PathFollowingController_SS_2/FlightOnSphere (Traction)/FlightPathLoopTraction ==
  Ft_set : Inport
  F_a_B_est : Inport  Port=2  PortDimensions=[3,1]
  StateEstimation_Bus : Inport  Port=3
  nu_chi : Inport  Port=4
  nu_gamma : Inport  Port=5
  Enable : EnablePort  StatesWhenEnabling=reset
  Bus Selector : BusSelector  OutputSignals=pos_G_O_m,pathangles_k,v_k_B,airdata,mu_a
  Delay : Delay  DelayLength=1  InitialConditionSource=Input port
      settings: InputPortMap=u0,p4
  Delay1 : Delay  DelayLength=1  InitialConditionSource=Input port
      settings: InputPortMap=u0,p4
  Delay{2..5} (4 alike) : Delay  DelayLength=1
  Demux : Demux  Outputs=2
  Demux1 : Demux  Outputs=2
  Demux2 : Demux  Outputs=2
  EstimatePlantResponse : Subsystem
  MATLAB Function : MATLAB Function  TreatAsAtomicUnit=on
  Mux : Mux  Inputs=2
  Saturation : Saturate  UpperLimit=constr.alpha_a_max  LowerLimit=constr.alpha_a_min
  Sum{,1..3} (4 alike) : Sum  Inputs=|+-
  inversionPathDynamics : MATLAB Function  TreatAsAtomicUnit=on
  mu_a_c_traction : Outport  PortDimensions=1
  alpha_rq : Outport  Port=2  PortDimensions=1
  wires:
  Bus Selector/5 -> Delay/2  "<mu_a>"
  F_a_B_est/1 -> inversionPathDynamics/4(F_a_B_est)
  Demux1/1 -> inversionPathDynamics/6(chi_k)
  inversionPathDynamics/1(mu_a) -> Delay/1, mu_a_c_traction/1
  Mux/1 -> Demux/1
  Demux/2 -> inversionPathDynamics/3(nu_gamma_k)
  Demux/1 -> inversionPathDynamics/2(nu_chi_k)
  inversionPathDynamics/2(mu_k_c) -> EstimatePlantResponse/3(mu_k_sat)
  inversionPathDynamics/3(alpha_rq) -> Saturation/1
  Saturation/1 -> alpha_rq/1, EstimatePlantResponse/2(alpha_rq)
  inversionPathDynamics/4(dphi) -> EstimatePlantResponse/1(dphi)
  Delay1/1 -> inversionPathDynamics/10(L_rq_old)
  Delay/1 -> inversionPathDynamics/11(mu_a_old)
  MATLAB Function/1(L_rq) -> Delay1/2
  inversionPathDynamics/5(L_rq) -> Delay1/1
  Demux1/2 -> inversionPathDynamics/7(gamma_k)
  StateEstimation_Bus/1 -> EstimatePlantResponse/5(StateEstimation_Bus), Bus Selector/1
  Bus Selector/4 -> inversionPathDynamics/9(airdata), MATLAB Function/1(airdata)  "<airdata>"
  Bus Selector/2 -> Demux1/1  "<pathangles_k>"
  Bus Selector/3 -> inversionPathDynamics/8(v_k_B)  "<v_k_B>"
  Bus Selector/1 -> inversionPathDynamics/5(pos_O)  "<pos_G_O_m>"
  Delay5/1 -> Sum3/1
  nu_chi/1 -> Sum/1
  Sum3/1 -> Sum/2
  Delay4/1 -> Sum2/2
  Delay3/1 -> Sum3/2
  Demux2/2 -> Delay4/1
  Sum1/1 -> Mux/2, Delay2/1
  Sum/1 -> Mux/1, Delay5/1
  Delay2/1 -> Sum2/1
  EstimatePlantResponse/1(pathAngleRate) -> Demux2/1
  nu_gamma/1 -> Sum1/1
  Demux2/1 -> Delay3/1
  Sum2/1 -> Sum1/2
  Ft_set/1 -> EstimatePlantResponse/4(Ft), inversionPathDynamics/1(Ft_set)

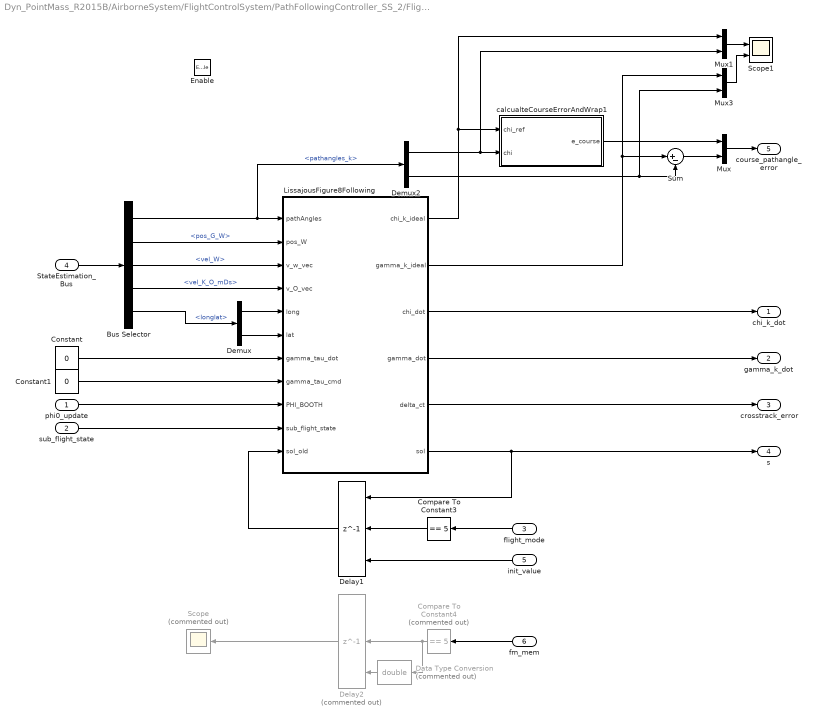
== system Dyn_PointMass_R2015B/AirborneSystem/FlightControlSystem/PathFollowingController_SS_2/FlightOnSphere (Traction)/Navigator ==
  phi0_update : Inport
  sub_flight_state : Inport  Port=2
  flight_mode : Inport  Port=3
  StateEstimation_Bus : Inport  Port=4
  init_value : Inport  Port=5
  fm_mem : Inport  Port=6
  Enable : EnablePort  StatesWhenEnabling=reset
  Bus Selector : BusSelector  OutputSignals=pathangles_k,pos_G_W,vel_W,vel_K_O_mDs,longlat
  Compare To Constant3 : simulink/Logic and Bit Operations/Compare To Constant  relop===  const=5  OutDataTypeStr=boolean
  Compare To Constant4 : simulink/Logic and Bit Operations/Compare To Constant  Commented=on  relop===  const=5  OutDataTypeStr=boolean
  Constant : Constant  Value=0
  Constant1 : Constant  Value=0
  Data Type Conversion : DataTypeConversion  Commented=on  OutDataTypeStr=double
  Delay1 : Delay  DelayLength=1  InitialConditionSource=Input port  InitialCondition=pi/2  ExternalReset=Rising
      settings: InputPortMap=u0,r5,p4
  Delay2 : Delay  Commented=on  DelayLength=1  InitialConditionSource=Input port  InitialCondition=pi/2  ExternalReset=Rising
      settings: InputPortMap=u0,r5,p4
  Demux : Demux  Outputs=2
  Demux2 : Demux  Outputs=2
  LissajousFigure8Following : MATLAB Function  TreatAsAtomicUnit=on
  Mux : Mux  Inputs=2
  Mux1 : Mux  Inputs=2
  Mux3 : Mux  Inputs=2
  Scope : Scope  Commented=on
  Scope1 : Scope  NumInputPorts=2
  Sum : Sum  Inputs=|+-
  calcualteCourseErrorAndWrap1 : MATLAB Function  TreatAsAtomicUnit=on
  chi_k_dot : Outport  PortDimensions=1
  gamma_k_dot : Outport  Port=2  PortDimensions=1
  crosstrack_error : Outport  Port=3
  s : Outport  Port=4  PortDimensions=1  InitialOutput=0
  course_pathangle_error : Outport  Port=5
  wires:
  Mux3/1 -> Scope1/2
  Mux1/1 -> Scope1/1
  Delay1/1 -> LissajousFigure8Following/11(sol_old)
  LissajousFigure8Following/6(sol) -> s/1, Delay1/1
  Bus Selector/4 -> LissajousFigure8Following/4(v_O_vec)  "<vel_K_O_mDs>"
  Demux/1 -> LissajousFigure8Following/5(long)
  calcualteCourseErrorAndWrap1/1(e_course) -> Mux/1
  LissajousFigure8Following/1(chi_k_ideal) -> calcualteCourseErrorAndWrap1/1(chi_ref), Mux1/1
  LissajousFigure8Following/2(gamma_k_ideal) -> Sum/1, Mux3/1
  Demux2/1 -> Mux1/2, calcualteCourseErrorAndWrap1/2(chi)
  Demux2/2 -> Mux3/2, Sum/2
  Mux/1 -> course_pathangle_error/1
  LissajousFigure8Following/4(gamma_dot) -> gamma_k_dot/1
  LissajousFigure8Following/3(chi_dot) -> chi_k_dot/1
  Sum/1 -> Mux/2
  Demux/2 -> LissajousFigure8Following/6(lat)
  LissajousFigure8Following/5(delta_ct) -> crosstrack_error/1
  StateEstimation_Bus/1 -> Bus Selector/1
  Bus Selector/2 -> LissajousFigure8Following/2(pos_W)  "<pos_G_W>"
  Bus Selector/5 -> Demux/1  "<longlat>"
  Bus Selector/1 -> Demux2/1, LissajousFigure8Following/1(pathAngles)  "<pathangles_k>"
  flight_mode/1 -> Compare To Constant3/1
  phi0_update/1 -> LissajousFigure8Following/9(PHI_BOOTH)
  Compare To Constant3/1 -> Delay1/2
  init_value/1 -> Delay1/3
  Constant/1 -> LissajousFigure8Following/7(gamma_tau_dot)
  Bus Selector/3 -> LissajousFigure8Following/3(v_w_vec)  "<vel_W>"
  Constant1/1 -> LissajousFigure8Following/8(gamma_tau_cmd)
  Delay2/1 -> Scope/1
  Compare To Constant4/1 -> Delay2/2, Data Type Conversion/1
  fm_mem/1 -> Compare To Constant4/1
  Data Type Conversion/1 -> Delay2/3
  sub_flight_state/1 -> LissajousFigure8Following/10(sub_flight_state)

== system Dyn_PointMass_R2015B/AirborneSystem/FlightControlSystem/PathFollowingController_SS_2/FlightOnSphere (Traction)/Pcontroller_ChiGamma_Traction ==
  course_pathangle_error : Inport
  Demux : Demux  Outputs=2
  Kp : Gain  Gain=params.Kp_gamma_k_traction  Multiplication=Matrix(K*u)
  Kp1 : Gain  Gain=params.Kp_chi_k_traction  Multiplication=Matrix(K*u)
  Chi_cntr : Outport
  Gamma_cntr : Outport  Port=2
  wires:
  Kp1/1 -> Chi_cntr/1
  Kp/1 -> Gamma_cntr/1
  course_pathangle_error/1 -> Demux/1
  Demux/2 -> Kp/1
  Demux/1 -> Kp1/1

== system Dyn_PointMass_R2015B/Environment_SS_3/Windshear/Wind Shear Model/wind_field_calc/Length Conversion ==
  in : Inport
  Unit Conversion : UnitConversion
  out : Outport
  wires:
  Unit Conversion/1 -> out/1
  in/1 -> Unit Conversion/1

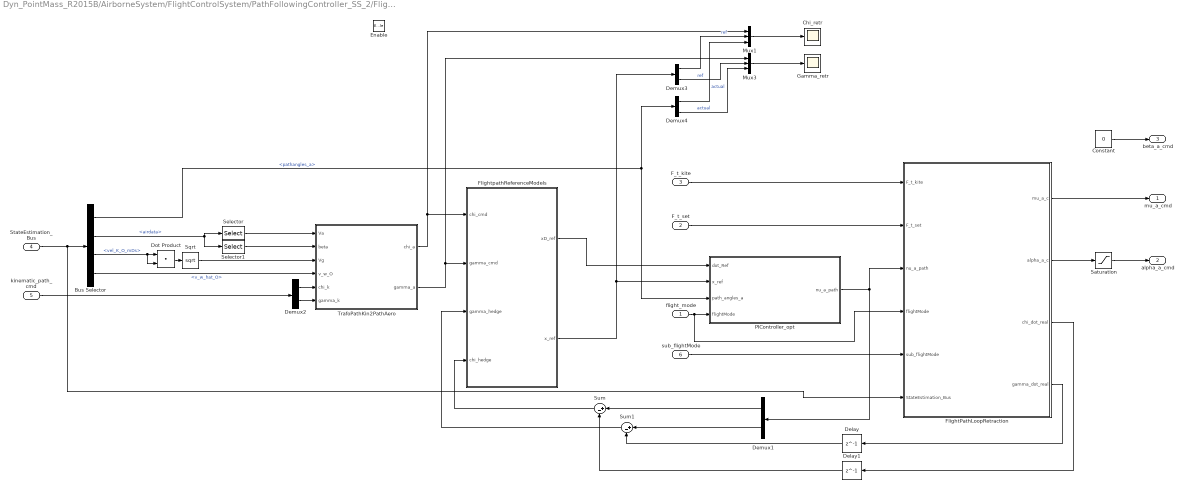
== system Dyn_PointMass_R2015B/AirborneSystem/FlightControlSystem/PathFollowingController_SS_2/FlightOnFlatEarth (Retraction&Loitering)/CalculateAttitudeCmds/FlightPathLoopRetraction_Aerodynamic ==
  flight_mode : Inport
  F_t_set : Inport  Port=2
  F_t_kite : Inport  Port=3
  StateEstimation_Bus : Inport  Port=4
  kinematic_path_cmd : Inport  Port=5
  sub_flightMode : Inport  Port=6
  Enable : EnablePort  StatesWhenEnabling=reset
  Bus Selector : BusSelector  OutputSignals=pathangles_a,airdata,vel_K_O_mDs,v_w_hat_O
  Chi_retr : Scope
  Constant : Constant  Value=0
  Delay : Delay  DelayLength=1
  Delay1 : Delay  DelayLength=1
  Demux{1..4} (4 alike) : Demux  Outputs=2
  Dot Product : DotProduct  InputSameDT=on  OutDataTypeStr=Inherit: Inherit via internal rule
  FlightPathLoopRetraction : Subsystem
  FlightpathReferenceModels : Subsystem
  Gamma_retr : Scope
  Mux1 : Mux  Inputs=3
  Mux3 : Mux  Inputs=3
  PIController_opt : Subsystem
  Saturation : Saturate  UpperLimit=constr.alpha_a_max  LowerLimit=constr.alpha_a_min
  Selector : Selector  InputPortWidth=3  IndexOptions=Index vector (dialog)  Indices=1  OutputSizes=1
  Selector1 : Selector  InputPortWidth=3  IndexOptions=Index vector (dialog)  Indices=3  OutputSizes=1
  Sqrt : Sqrt  SaturateOnIntegerOverflow=on
  Sum : Sum  Inputs=|+-
  Sum1 : Sum  Inputs=|+-
  TrafoPathKin2PathAero : MATLAB Function  TreatAsAtomicUnit=on
  mu_a_cmd : Outport
  alpha_a_cmd : Outport  Port=2
  beta_a_cmd : Outport  Port=3
  wires:
  StateEstimation_Bus/1 -> Bus Selector/1, FlightPathLoopRetraction/6(StateEstimation_Bus)
  Bus Selector/1 -> Demux4/1, PIController_opt/3(path_angles_a)  "<pathangles_a>"
  Bus Selector/3 -> Dot Product/2, Dot Product/1  "<vel_K_O_mDs>"
  Bus Selector/2 -> Selector1/1, Selector/1  "<airdata>"
  F_t_kite/1 -> FlightPathLoopRetraction/1(F_t_kite)
  Mux3/1 -> Gamma_retr/1
  Mux1/1 -> Chi_retr/1
  Demux4/1 -> Mux1/3  "actual"
  Demux3/2 -> Mux3/2  "ref"
  Demux4/2 -> Mux3/3  "actual"
  Demux3/1 -> Mux1/2  "ref"
  Demux2/2 -> TrafoPathKin2PathAero/6(gamma_k)
  FlightpathReferenceModels/2(x_ref) -> Demux3/1, PIController_opt/2(x_ref)
  Demux2/1 -> TrafoPathKin2PathAero/5(chi_k)
  FlightPathLoopRetraction/1(mu_a_c) -> mu_a_cmd/1
  FlightpathReferenceModels/1(xD_ref) -> PIController_opt/1(dot_Ref)
  Constant/1 -> beta_a_cmd/1
  FlightPathLoopRetraction/3(chi_dot_real) -> Delay1/1
  PIController_opt/1(nu_a_path) -> FlightPathLoopRetraction/3(nu_a_path), Demux1/1
  Saturation/1 -> alpha_a_cmd/1
  FlightPathLoopRetraction/2(alpha_a_c) -> Saturation/1
  Dot Product/1 -> Sqrt/1
  Sqrt/1 -> TrafoPathKin2PathAero/3(Vg)
  Selector/1 -> TrafoPathKin2PathAero/1(Va)
  TrafoPathKin2PathAero/1(chi_a) -> Mux1/1, FlightpathReferenceModels/1(chi_cmd)
  TrafoPathKin2PathAero/2(gamma_a) -> Mux3/1, FlightpathReferenceModels/2(gamma_cmd)
  Selector1/1 -> TrafoPathKin2PathAero/2(beta)
  F_t_set/1 -> FlightPathLoopRetraction/2(F_t_set)
  kinematic_path_cmd/1 -> Demux2/1
  Bus Selector/4 -> TrafoPathKin2PathAero/4(v_w_O)  "<v_w_hat_O>"
  flight_mode/1 -> PIController_opt/4(flightMode), FlightPathLoopRetraction/4(flightMode)
  FlightPathLoopRetraction/4(gamma_dot_real) -> Delay/1
  Demux1/1 -> Sum/1
  Demux1/2 -> Sum1/1
  Sum/1 -> FlightpathReferenceModels/4(chi_hedge)
  Sum1/1 -> FlightpathReferenceModels/3(gamma_hedge)
  Delay/1 -> Sum1/2
  Delay1/1 -> Sum/2
  sub_flightMode/1 -> FlightPathLoopRetraction/5(sub_flightMode)

== system Dyn_PointMass_R2015B/AirborneSystem/FlightControlSystem/PathFollowingController_SS_2/FlightOnFlatEarth (Retraction&Loitering)/GuidanceFlatEarth/LoiteringGuidance ==
  flightMode : Inport
  pos_G_O_m : Inport  Port=2
  vel_K_O_mDs : Inport  Port=3
  pathangles_k : Inport  Port=4
  pos_W : Inport  Port=5
  reset_flag : Inport  Port=6
  Compare To Constant3 : simulink/Logic and Bit Operations/Compare To Constant  relop===  const=1  OutDataTypeStr=boolean
  Constant1 : Constant  Value=ENVMT.windDirection_rad
  Constant3 : Constant  Value=0
  Delay : Delay  DelayLength=1  InitialConditionSource=Input port  ExternalReset=Rising
      settings: InputPortMap=u0,r5,p4
  Delay1 : Delay  DelayLength=1  InitialConditionSource=Input port  ExternalReset=Rising
      settings: InputPortMap=u0,r5,p4
  Dot Product : DotProduct  InputSameDT=on  OutDataTypeStr=Inherit: Inherit via internal rule
  Gain1 : Gain  Gain=-1
  Loiter : Stateflow chart  TreatAsAtomicUnit=on  mask{kp_course_init=loiterStates.kp_delta_course, pos_OLoiter_W=loiterStates.pos_OLoiter_W, R_init_loiter=loiterStates.R, validTransReg_start=loiterStates.validTransReg_start, validTransReg_end=loiterStates.validTransReg_end}
  Mux : Mux  Inputs=2
  Selector1 : Selector  InputPortWidth=2  IndexOptions=Index vector (dialog)  Indices=1  OutputSizes=1
  Selector2 : Selector  InputPortWidth=3  IndexOptions=Index vector (dialog)  Indices=2  OutputSizes=1
  Selector3 : Selector  InputPortWidth=3  IndexOptions=Index vector (dialog)  Indices=1  OutputSizes=1
  Selector4 : Selector  InputPortWidth=3  IndexOptions=Index vector (dialog)  Indices=3  OutputSizes=1
  Sqrt : Sqrt  SaturateOnIntegerOverflow=on
  Subsystem : Subsystem
  Terminator1 : Terminator
  path_k_cmds : Outport
  valid_transition_region : Outport  Port=2
  wires:
  pathangles_k/1 -> Selector1/1
  Mux/1 -> path_k_cmds/1
  Selector1/1 -> Delay/3
  Selector4/1 -> Gain1/1
  Compare To Constant3/1 -> Delay1/2
  pos_W/1 -> Selector2/1, Selector3/1
  Dot Product/1 -> Sqrt/1
  Sqrt/1 -> Loiter/4(Vk)
  Delay1/1 -> Delay1/1, Subsystem/2(h_cmd)
  Loiter/1(course_des) -> Mux/1
  vel_K_O_mDs/1 -> Subsystem/1(v_k_O), Dot Product/1, Dot Product/2
  pos_G_O_m/1 -> Subsystem/3(h), Selector4/1
  Selector3/1 -> Loiter/3(p_x_W)
  Gain1/1 -> Delay1/3
  Subsystem/1(gamma_k_cmd) -> Mux/2
  Delay/1 -> Loiter/2(course_k), Delay/1
  Selector2/1 -> Loiter/1(p_y_W)
  Loiter/2(valid_transition_region_flag) -> valid_transition_region/1
  reset_flag/1 -> Loiter/5(reset_flag)
  Constant1/1 -> Loiter/6(windDir)
  Constant3/1 -> Delay/2
  flightMode/1 -> Compare To Constant3/1
  Loiter/3(e_track) -> Terminator1/1

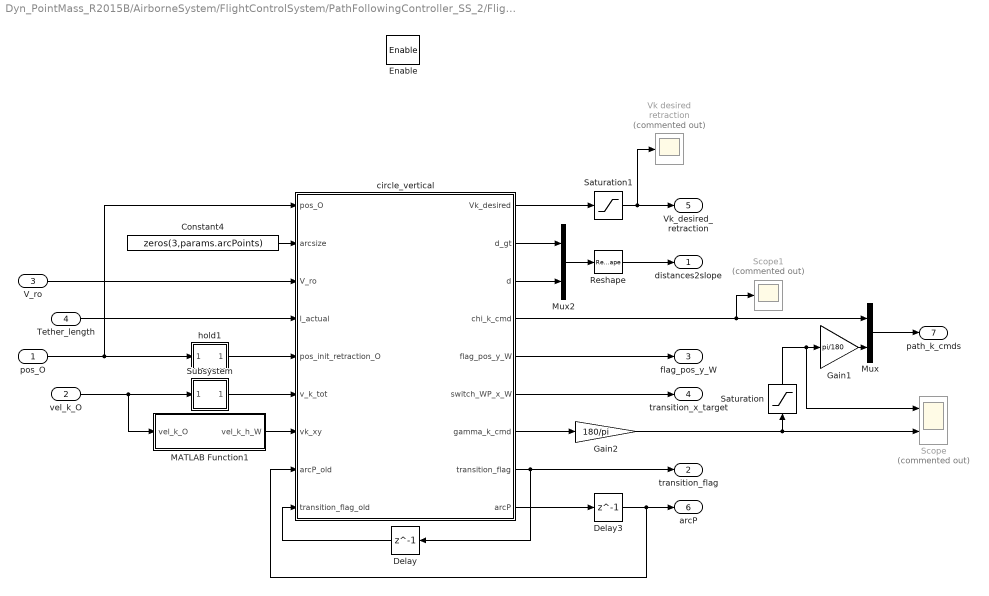
== system Dyn_PointMass_R2015B/AirborneSystem/FlightControlSystem/PathFollowingController_SS_2/FlightOnFlatEarth (Retraction&Loitering)/GuidanceFlatEarth/Retraction_Nav ==
  pos_O : Inport
  vel_k_O : Inport  Port=2
  V_ro : Inport  Port=3
  Tether_length : Inport  Port=4
  Enable : EnablePort  StatesWhenEnabling=reset
  Constant4 : Constant  Value=zeros(3,params.arcPoints)
  Delay : Delay  DelayLength=1
  Delay3 : Delay  DelayLength=1  InitialCondition=zeros(3,params.arcPoints)
  Gain1 : Gain  Gain=pi/180
  Gain2 : Gain  Gain=180/pi
  MATLAB Function1 : MATLAB Function  TreatAsAtomicUnit=on
  Mux : Mux  Inputs=2
  Mux2 : Mux  Inputs=2
  Reshape : Reshape  OutputDimensionality=Row vector (2-D)
  Saturation : Saturate  UpperLimit=constr.gamma_max_retraction  LowerLimit=constr.gamma_min_retraction
  Saturation1 : Saturate  UpperLimit=300  LowerLimit=0
  Scope : Scope  Commented=on  NumInputPorts=2
  Scope1 : Scope  Commented=on
  Subsystem : Subsystem
      mask Display: disp('norm()')
  Vk desired retraction : Scope  Commented=on
  circle_vertical : MATLAB Function  TreatAsAtomicUnit=on
  hold1 : Subsystem
      mask Display: disp('hold()', 'texmode','on')
  distances2slope : Outport
  transition_flag : Outport  Port=2
  flag_pos_y_W : Outport  Port=3
  transition_x_target : Outport  Port=4
  Vk_desired_retraction : Outport  Port=5
  arcP : Outport  Port=6
  path_k_cmds : Outport  Port=7  PortDimensions=[2,1]
  wires:
  circle_vertical/7(gamma_k_cmd) -> Gain2/1
  circle_vertical/8(transition_flag) -> Delay/1, transition_flag/1
  MATLAB Function1/1(vel_k_h_W) -> circle_vertical/7(vk_xy)
  circle_vertical/2(d_gt) -> Mux2/1
  Mux2/1 -> Reshape/1
  circle_vertical/4(chi_k_cmd) -> Mux/1, Scope1/1
  Gain1/1 -> Mux/2
  hold1/1(Out1) -> circle_vertical/5(pos_init_retraction_O)
  circle_vertical/3(d) -> Mux2/2
  vel_k_O/1 -> Subsystem/1(In1), MATLAB Function1/1(vel_k_O)
  Saturation/1 -> Gain1/1, Scope/1
  Mux/1 -> path_k_cmds/1
  Delay/1 -> circle_vertical/9(transition_flag_old)
  Reshape/1 -> distances2slope/1
  circle_vertical/5(flag_pos_y_W) -> flag_pos_y_W/1
  circle_vertical/6(switch_WP_x_W) -> transition_x_target/1
  Gain2/1 -> Saturation/1, Scope/2
  Tether_length/1 -> circle_vertical/4(l_actual)
  V_ro/1 -> circle_vertical/3(V_ro)
  circle_vertical/1(Vk_desired) -> Saturation1/1
  Saturation1/1 -> Vk desired retraction/1, Vk_desired_retraction/1
  Constant4/1 -> circle_vertical/2(arcsize)
  circle_vertical/9(arcP) -> Delay3/1
  Delay3/1 -> circle_vertical/8(arcP_old), arcP/1
  pos_O/1 -> circle_vertical/1(pos_O), hold1/1(In1)
  Subsystem/1(Out1) -> circle_vertical/6(v_k_tot)

== system Dyn_PointMass_R2015B/AirborneSystem/FlightControlSystem/PathFollowingController_SS_2/FlightOnSphere (Traction)/FlightPathLoopTraction/EstimatePlantResponse ==
  dphi : Inport
  alpha_rq : Inport  Port=2
  mu_k_sat : Inport  Port=3
  Ft : Inport  Port=4
  StateEstimation_Bus : Inport  Port=5
  Bus Selector : BusSelector  OutputSignals=pathangles_k,pos_G_O_m,v_k_B,airdata
  Demux : Demux  Outputs=2
  MATLAB Function : MATLAB Function  TreatAsAtomicUnit=on
  Mux : Mux  Inputs=3
  Mux4 : Mux  Inputs=2
  Selector : Selector  InputPortWidth=3  IndexOptions=Index vector (dialog)  Indices=1  OutputSizes=1
  Selector1 : Selector  InputPortWidth=3  IndexOptions=Index vector (dialog)  Indices=3  OutputSizes=1
  pathAngleRate : Outport
  wires:
  MATLAB Function/2(gamma_dot_real) -> Mux4/2
  Mux4/1 -> pathAngleRate/1
  MATLAB Function/1(chi_dot_real) -> Mux4/1
  dphi/1 -> MATLAB Function/2(dphi)
  Demux/1 -> MATLAB Function/4(chi_k)
  Demux/2 -> MATLAB Function/5(gamma_k)
  Ft/1 -> MATLAB Function/1(F_t)
  mu_k_sat/1 -> MATLAB Function/3(mu_k)
  StateEstimation_Bus/1 -> Bus Selector/1
  Bus Selector/2 -> MATLAB Function/6(pos_O)  "<pos_G_O_m>"
  Bus Selector/4 -> Selector1/1, Selector/1  "<airdata>"
  Bus Selector/3 -> MATLAB Function/7(v_k_B)  "<v_k_B>"
  Bus Selector/1 -> Demux/1  "<pathangles_k>"
  Selector/1 -> Mux/1
  Selector1/1 -> Mux/3
  alpha_rq/1 -> Mux/2
  Mux/1 -> MATLAB Function/8(airdata)
